simulink model "ANN_Simulation"  (R2024a)
settings: Solver=VariableStepAuto  StartTime=0.0  StopTime=5  RelTol=1e-3
undefined symbols (not defined in the file or in its folder): B, J, Ls, p, Rs, samplingTime, Sm
libraries: slpidlib x1
settings Model: Creator=anugr  LastModifiedBy=anugr
settings DataIOCC: ReturnWorkspaceOutputs=off

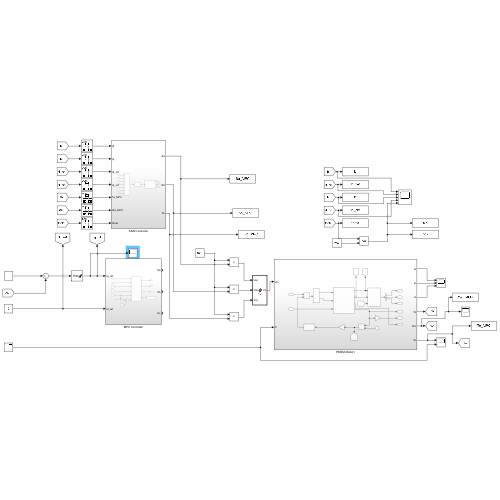
[thumbnail: Simulink's stored preview of the top-level diagram]
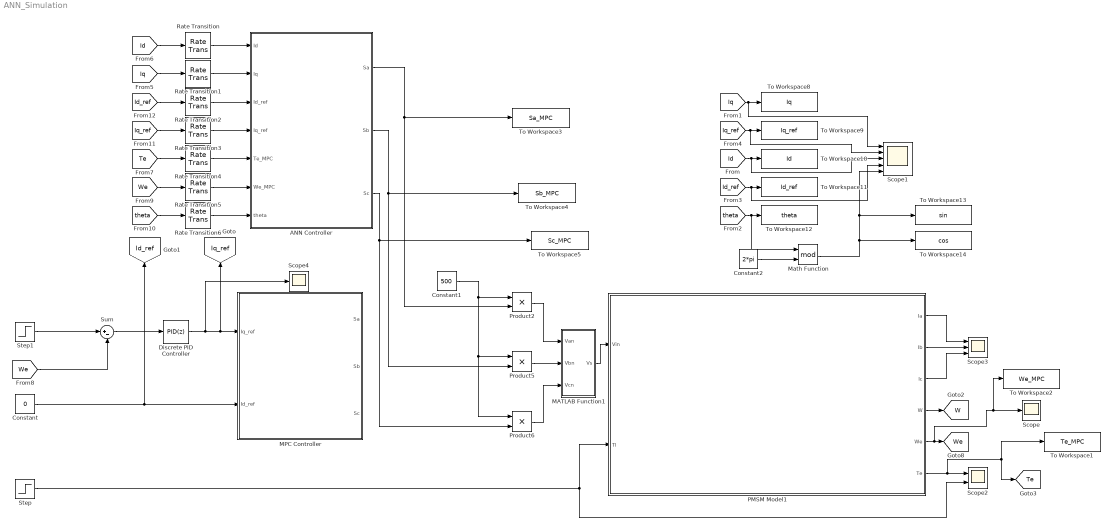
== system ANN_Simulation ==
  ANN Controller : Subsystem
  Constant : Constant  Value=0
  Constant1 : Constant  Value=500
  Constant2 : Constant  Value=2*pi
  Discrete PID Controller : slpidlib/PID Controller  Controller=PID  Form=Parallel  TimeDomain=Discrete-time  UseExternalTs=off  SampleTime=-1  IntegratorMethod=Forward Euler  FilterMethod=Forward Euler  ControllerParametersSource=internal  P=10  I=1  UseKiTs=off  D=1  UseExternalDerivativeSource=off  N=100  UseFilter=on  TunerSelectOption=Transfer Function Based (PID Tuner App)  InitialConditionSource=internal  InitialConditionForIntegrator=0  InitialConditionForFilter=0  DifferentiatorICPrevScaledInput=0  ExternalReset=none  TrackingMode=off  Kt=1  LimitOutput=on  SatLimitsSource=internal  UpperSaturationLimit=20  LowerSaturationLimit=-20  LinearizeAsGain=on  AntiWindupMode=clamping  Kb=1  LimitIntegrator=off  UpperIntegratorSaturationLimit=inf  LowerIntegratorSaturationLimit=-inf  POutMin=[]  POutMax=[]  IOutMin=[]  IOutMax=[]  DOutMin=[]  DOutMax=[]  NOutMin=[]  NOutMax=[]  SumOutMin=[]  SumOutMax=[]  SaturationOutMin=[]  SaturationOutMax=[]  PParamMin=[]  PParamMax=[]  IParamMin=[]  IParamMax=[]  DParamMin=[]  DParamMax=[]  NParamMin=[]  NParamMax=[]  KbParamMin=[]  KbParamMax=[]  KtParamMin=[]  KtParamMax=[]  KbOutMin=[]  KbOutMax=[]  KtOutMin=[]  KtOutMax=[]  IntegratorOutMin=[]  IntegratorOutMax=[]  FilterOutMin=[]  FilterOutMax=[]  SumI1OutMin=[]  SumI1OutMax=[]  SumI2OutMin=[]  SumI2OutMax=[]  SumI3OutMin=[]  SumI3OutMax=[]  SumI4OutMin=[]  SumI4OutMax=[]  SumDOutMin=[]  SumDOutMax=[]  DifferentiatorOutMin=[]  DifferentiatorOutMax=[]  FilterDiffOutCoefMin=[]  FilterDiffOutCoefMax=[]  ReciprocalOutMin=[]  ReciprocalOutMax=[]  SumDenOutMin=[]  SumDenOutMax=[]  SumNumOutMin=[]  SumNumOutMax=[]  DivideOutMin=[]  DivideOutMax=[]  UdiffTsProdOutMin=[]  UdiffTsProdOutMax=[]  NTsProdOutMin=[]  NTsProdOutMax=[]  UintegralTsProdOutMin=[]  UintegralTsProdOutMax=[]  UngainTsProdOutMin=[]  UngainTsProdOutMax=[]  ClampingZeroOutDataTypeStr=Inherit: Inherit via back propagation  ClampingZeroOutMin=[]  ClampingZeroOutMax=[]  FilterDenConstantOutDataTypeStr=Inherit: Inherit via back propagation  FilterDenConstantOutMin=[]  FilterDenConstantOutMax=[]  PCopyOutDataTypeStr=Inherit: Inherit via back propagation  PCopyOutMin=[]  PCopyOutMax=[]  NCopyOutDataTypeStr=Inherit: Inherit via back propagation  NCopyOutMin=[]  NCopyOutMax=[]  IntegratorContinuousStateAttributes=''  IntegratorStateMustResolveToSignalObject=off  IntegratorRTWStateStorageClass=Auto  FilterContinuousStateAttributes=''  FilterStateMustResolveToSignalObject=off  FilterRTWStateStorageClass=Auto  ParallelPVariant=InternalParameters  IdealPVariant=Disabled  IVariant=InternalParameters  DVariant=InternalParameters  IntegratorVariant=Discrete  SatVariant=Enabled  AWVariant=DiscClampingParallel  PCopyVariant=Disabled  TRVariant=Disabled  FdbkBlocksVariant=Forward  IdealPFdbkVariant=Disabled  SatFdbkVariant=Disabled  DerivativeFilterVariant=ForwardEulerFilter  NVariant=InternalParameters  NCopyVariant=Disabled  FilterICVariant=InternalICsFilter  IntegratorICVariant=InternalICs  ExternalResetVariant=Disabled  TRSumVariant=Passthrough  SumFdbkVariant=Disabled  SumVariant=Sum_PID  TsampFilterVariant=InternalTs  TsampNgainVariant=Passthrough  TsampIntegralVariant=Disabled_SignalSpec  ExternalSaturationOutDataTypeStr=Inherit: Same as second input  DerivativeSourceVariant=ErrorSignal
  MATLAB Function1 : MATLAB Function  TreatAsAtomicUnit=on
  MPC Controller : Subsystem
  Math Function : Math  Operator=mod
  PMSM Model1 : Subsystem
  Product2 : Product
  Product5 : Product
  Product6 : Product
  Rate Transition{,1..6} (7 alike) : RateTransition  OutPortSampleTime=5e-5
  Scope : Scope
  Scope1 : Scope  NumInputPorts=5
  Scope2 : Scope  NumInputPorts=2
  Scope3 : Scope  NumInputPorts=3
  Scope4 : Scope
  Step : Step  Time=2.5  After=5  SampleTime=0
  Step1 : Step  Time=0  After=200  SampleTime=0
  Sum : Sum  Inputs=|+-
  To Workspace1 : ToWorkspace  VariableName=Te_MPC  SampleTime=samplingTime*1e-6
      settings: Save2DSignal=2-D array (concatenate along first dimension)
  To Workspace10 : ToWorkspace  VariableName=Id  SampleTime=samplingTime*1e-6
      settings: Save2DSignal=2-D array (concatenate along first dimension)
  To Workspace11 : ToWorkspace  VariableName=Id_ref  SampleTime=samplingTime*1e-6
      settings: Save2DSignal=2-D array (concatenate along first dimension)
  To Workspace12 : ToWorkspace  VariableName=theta  SampleTime=samplingTime*1e-6
      settings: Save2DSignal=2-D array (concatenate along first dimension)
  To Workspace13 : ToWorkspace  VariableName=sin  SampleTime=samplingTime*1e-6
      settings: Save2DSignal=2-D array (concatenate along first dimension)
  To Workspace14 : ToWorkspace  VariableName=cos  SampleTime=samplingTime*1e-6
      settings: Save2DSignal=2-D array (concatenate along first dimension)
  To Workspace2 : ToWorkspace  VariableName=We_MPC  SampleTime=samplingTime*1e-6
      settings: Save2DSignal=2-D array (concatenate along first dimension)
  To Workspace3 : ToWorkspace  VariableName=Sa_MPC  SampleTime=samplingTime*1e-6
      settings: Save2DSignal=2-D array (concatenate along first dimension)
  To Workspace4 : ToWorkspace  VariableName=Sb_MPC  SampleTime=samplingTime*1e-6
      settings: Save2DSignal=2-D array (concatenate along first dimension)
  To Workspace5 : ToWorkspace  VariableName=Sc_MPC  SampleTime=samplingTime*1e-6
      settings: Save2DSignal=2-D array (concatenate along first dimension)
  To Workspace8 : ToWorkspace  VariableName=Iq  SampleTime=samplingTime*1e-6
      settings: Save2DSignal=2-D array (concatenate along first dimension)
  To Workspace9 : ToWorkspace  VariableName=Iq_ref  SampleTime=samplingTime*1e-6
      settings: Save2DSignal=2-D array (concatenate along first dimension)
  tag scope: Id_ref=global, Iq_ref=global, Te=global, W=global, We=global
  wires:
  [Iq_ref] -> Scope1/2, To Workspace9/1
  [Id] -> Scope1/3, To Workspace10/1
  Product6/1 -> MATLAB Function1/3(Vcn)
  Product5/1 -> MATLAB Function1/2(Vbn)
  Math Function/1 -> To Workspace14/1, To Workspace13/1, Scope1/5
  Constant2/1 -> Math Function/2
  PMSM Model1/2(Ib) -> Scope3/2
  Product2/1 -> MATLAB Function1/1(Van)
  PMSM Model1/1(Ia) -> Scope3/1
  PMSM Model1/5(We) -> To Workspace2/1, Scope/1, [We]
  [Iq] -> Scope1/1, To Workspace8/1
  [Id_ref] -> Scope1/4, To Workspace11/1
  [theta] -> Math Function/1, To Workspace12/1
  Sum/1 -> Discrete PID Controller/1
  Step1/1 -> Sum/1
  Discrete PID Controller/1 -> Scope4/1, [Iq_ref], MPC Controller/1(Iq_ref)
  Constant1/1 -> Product5/1, Product6/1, Product2/1
  PMSM Model1/4(W) -> [W]
  [We] -> Sum/2
  PMSM Model1/6(Te) -> To Workspace1/1, [Te], Scope2/1
  Constant/1 -> [Id_ref], MPC Controller/2(Id_ref)
  MATLAB Function1/1(Vs) -> PMSM Model1/1(Vin)
  Step/1 -> Scope2/2, PMSM Model1/2(Tl)
  PMSM Model1/3(Ic) -> Scope3/3
  [Iq] -> Rate Transition1/1
  [Id] -> Rate Transition/1
  [Te] -> Rate Transition4/1
  [We] -> Rate Transition5/1
  [theta] -> Rate Transition6/1
  [Iq_ref] -> Rate Transition3/1
  [Id_ref] -> Rate Transition2/1
  ANN Controller/1(Sa) -> Product2/2, To Workspace3/1
  ANN Controller/2(Sb) -> To Workspace4/1, Product5/2
  ANN Controller/3(Sc) -> Product6/2, To Workspace5/1
  Rate Transition/1 -> ANN Controller/1(Id)
  Rate Transition1/1 -> ANN Controller/2(Iq)
  Rate Transition2/1 -> ANN Controller/3(Id_ref)
  Rate Transition3/1 -> ANN Controller/4(Iq_ref)
  Rate Transition4/1 -> ANN Controller/5(Te_MPC)
  Rate Transition5/1 -> ANN Controller/6(We_MPC)
  Rate Transition6/1 -> ANN Controller/7(theta)

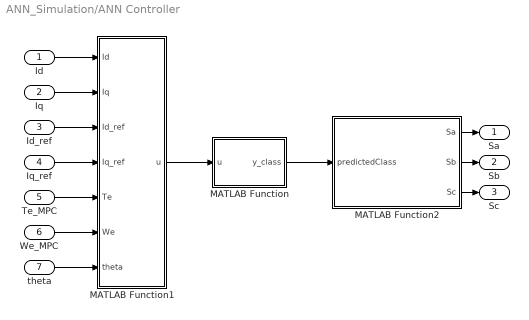
== system ANN_Simulation/ANN Controller ==
  Id : Inport
  Iq : Inport  Port=2
  Id_ref : Inport  Port=3
  Iq_ref : Inport  Port=4
  Te_MPC : Inport  Port=5
  We_MPC : Inport  Port=6
  theta : Inport  Port=7
  MATLAB Function : MATLAB Function  TreatAsAtomicUnit=on
  MATLAB Function1 : MATLAB Function  TreatAsAtomicUnit=on
  MATLAB Function2 : MATLAB Function  TreatAsAtomicUnit=on
  Sa : Outport
  Sb : Outport  Port=2
  Sc : Outport  Port=3
  wires:
  MATLAB Function2/3(Sc) -> Sc/1
  We_MPC/1 -> MATLAB Function1/6(We)
  Iq/1 -> MATLAB Function1/2(Iq)
  MATLAB Function2/1(Sa) -> Sa/1
  MATLAB Function/1(y_class) -> MATLAB Function2/1(predictedClass)
  theta/1 -> MATLAB Function1/7(theta)
  MATLAB Function1/1(u) -> MATLAB Function/1(u)
  Id/1 -> MATLAB Function1/1(Id)
  Te_MPC/1 -> MATLAB Function1/5(Te)
  MATLAB Function2/2(Sb) -> Sb/1
  Id_ref/1 -> MATLAB Function1/3(Id_ref)
  Iq_ref/1 -> MATLAB Function1/4(Iq_ref)

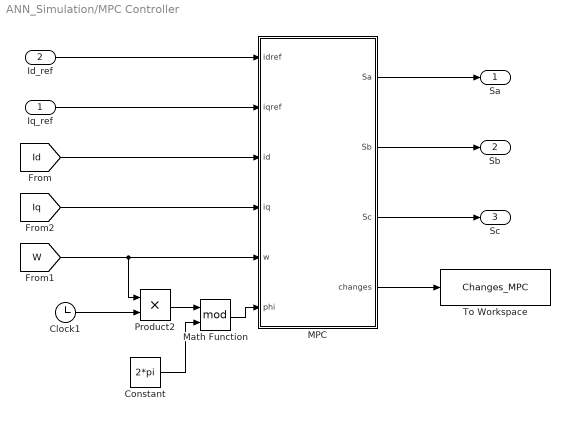
== system ANN_Simulation/MPC Controller ==
  Iq_ref : Inport
  Id_ref : Inport  Port=2
  Clock1 : Clock
  Constant : Constant  Value=2*pi
  MPC : MATLAB Function  TreatAsAtomicUnit=on
  Math Function : Math  Operator=mod
  Product2 : Product
  To Workspace : ToWorkspace  VariableName=Changes_MPC  SaveFormat=Timeseries  SampleTime=-1
  Sa : Outport
  Sb : Outport  Port=2
  Sc : Outport  Port=3
  wires:
  [Iq] -> MPC/4(iq)
  [W] -> MPC/5(w), Product2/1
  MPC/3(Sc) -> Sc/1
  [Id] -> MPC/3(id)
  Id_ref/1 -> MPC/1(idref)
  Iq_ref/1 -> MPC/2(iqref)
  Clock1/1 -> Product2/2
  MPC/2(Sb) -> Sb/1
  MPC/1(Sa) -> Sa/1
  MPC/4(changes) -> To Workspace/1
  Product2/1 -> Math Function/1
  Math Function/1 -> MPC/6(phi)
  Constant/1 -> Math Function/2

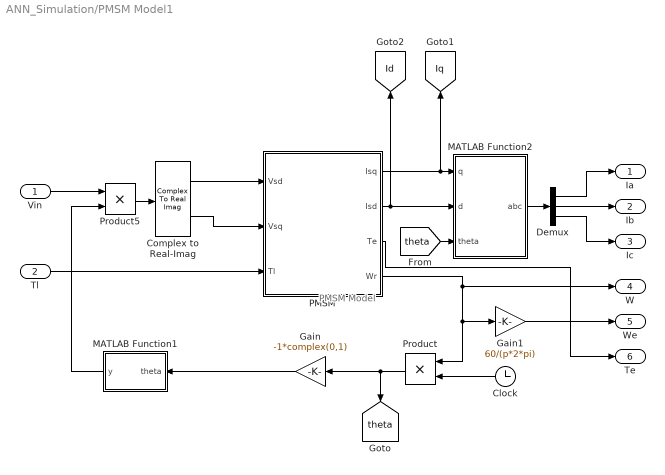
== system ANN_Simulation/PMSM Model1 ==
  note: PMSM Model
  Vin : Inport
  Tl : Inport  Port=2
  Clock : Clock
  Complex to Real-Imag : ComplexToRealImag
  Demux : Demux  Outputs=3
  Gain : Gain  Gain=-1*complex(0,1)
  Gain1 : Gain  Gain=60/(p*2*pi)
  MATLAB Function1 : MATLAB Function  TreatAsAtomicUnit=on
  MATLAB Function2 : MATLAB Function  TreatAsAtomicUnit=on
  PMSM : Subsystem
  Product : Product
  Product5 : Product
  Ia : Outport
  Ib : Outport  Port=2
  Ic : Outport  Port=3
  W : Outport  Port=4
  We : Outport  Port=5
  Te : Outport  Port=6
  tag scope: Id=global, Iq=global, theta=global
  wires:
  Tl/1 -> PMSM/3(Tl)
  PMSM/4(Wr) -> W/1, Gain1/1, Product/1
  Product/1 -> Gain/1, [theta]
  Demux/3 -> Ic/1
  Clock/1 -> Product/2
  PMSM/1(Isq) -> [Iq], MATLAB Function2/1(q)
  MATLAB Function1/1(y) -> Product5/2
  Complex to Real-Imag/1 -> PMSM/1(Vsd)
  PMSM/3(Te) -> Te/1
  PMSM/2(Isd) -> MATLAB Function2/2(d), [Id]
  Complex to Real-Imag/2 -> PMSM/2(Vsq)
  Product5/1 -> Complex to Real-Imag/1
  Gain/1 -> MATLAB Function1/1(theta)
  Demux/1 -> Ia/1
  MATLAB Function2/1(abc) -> Demux/1
  Vin/1 -> Product5/1
  Gain1/1 -> We/1
  Demux/2 -> Ib/1
  [theta] -> MATLAB Function2/3(theta)

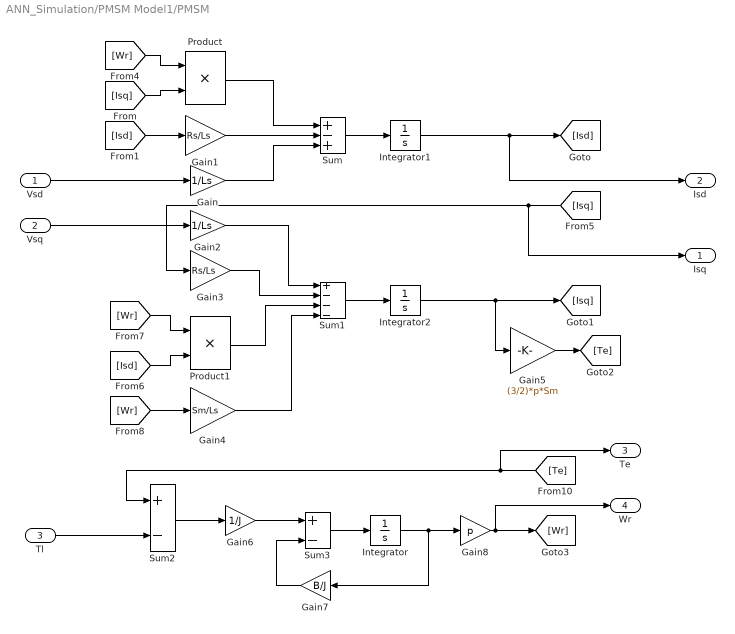
== system ANN_Simulation/PMSM Model1/PMSM ==
  Vsd : Inport
  Vsq : Inport  Port=2
  Tl : Inport  Port=3
  Gain : Gain  Gain=1/Ls
  Gain1 : Gain  Gain=Rs/Ls
  Gain2 : Gain  Gain=1/Ls
  Gain3 : Gain  Gain=Rs/Ls
  Gain4 : Gain  Gain=Sm/Ls
  Gain5 : Gain  Gain=(3/2)*p*Sm
  Gain6 : Gain  Gain=1/J
  Gain7 : Gain  Gain=B/J
  Gain8 : Gain  Gain=p
  Integrator : Integrator
  Integrator1 : Integrator
  Integrator2 : Integrator
  Product : Product
  Product1 : Product
  Sum : Sum  Inputs=+-+
  Sum1 : Sum  Inputs=+---
  Sum2 : Sum  Inputs=+-
  Sum3 : Sum  Inputs=+-
  Isq : Outport
  Isd : Outport  Port=2
  Te : Outport  Port=3
  Wr : Outport  Port=4
  wires:
  Gain5/1 -> [Te]
  [Wr] -> Gain4/1
  [Isq] -> Isq/1, Gain3/1
  [Te] -> Te/1, Sum2/1
  Integrator2/1 -> Gain5/1, [Isq]
  Gain6/1 -> Sum3/1
  Sum1/1 -> Integrator2/1
  Gain/1 -> Sum/3
  Integrator/1 -> Gain8/1, Gain7/1
  Tl/1 -> Sum2/2
  Gain8/1 -> Wr/1, [Wr]
  Gain2/1 -> Sum1/1
  Sum3/1 -> Integrator/1
  Vsd/1 -> Gain/1
  Sum2/1 -> Gain6/1
  [Isd] -> Product1/2
  Gain7/1 -> Sum3/2
  Gain3/1 -> Sum1/2
  Gain4/1 -> Sum1/4
  [Wr] -> Product/1
  [Isq] -> Product/2
  Product1/1 -> Sum1/3
  [Wr] -> Product1/1
  Product/1 -> Sum/1
  Gain1/1 -> Sum/2
  [Isd] -> Gain1/1
  Sum/1 -> Integrator1/1
  Vsq/1 -> Gain2/1
  Integrator1/1 -> Isd/1, [Isd]

== matlab function ANN_Simulation/ANN Controller/MATLAB Function1 ==
  data: Id input; u output; Iq input; Id_ref input; Iq_ref input; Te input; We input; theta input
function u = createANNInputs(Id, Iq, Id_ref, Iq_ref, Te, We, theta)
%#codegen
sinTheta = sin(theta);
cosTheta = cos(theta);
u = [Id; Iq; Id_ref; Iq_ref; Te; We; theta; sinTheta; cosTheta];
end

== matlab function ANN_Simulation/ANN Controller/MATLAB Function ==
  data: u input; y_class output
function y_class = runANN(u)
%#codegen
y = myANNFcn(u);         % ANN raw output (numClasses × 1)
[~, idx] = max(y);       % pick highest activation
y_class = idx - 1;       % convert to class label (0–7)
end

== matlab function ANN_Simulation/ANN Controller/MATLAB Function2 ==
  data: predictedClass input; Sa output; Sb output; Sc output
function [Sa, Sb, Sc] = classToSwitching(predictedClass)
%CLASSTOSWITCHING Converts ANN class output to 3-phase switching signals
%   Input:
%       predictedClass - scalar, integer class (0 to 7)
%   Outputs:
%       Sa, Sb, Sc    - switching signals (0 or 1)

    switch predictedClass
        case 0
            Sa = 0; Sb = 0; Sc = 0;
        case 1
            Sa = 1; Sb = 0; Sc = 0;
        case 2
            Sa = 1; Sb = 1; Sc = 0;
        case 3
            Sa = 0; Sb = 1; Sc = 0;
        case 4
            Sa = 0; Sb = 1; Sc = 1;
        case 5
            Sa = 0; Sb = 0; Sc = 1;
        case 6
            Sa = 1; Sb = 0; Sc = 1;
        case 7
            Sa = 1; Sb = 1; Sc = 1;
        otherwise
            error('Invalid class. Must be an integer from 0 to 7.');
    end
end

== matlab function ANN_Simulation/MPC Controller/MPC ==
  settings: updateMethod=DISCRETE
  data: idref input; Sa output; iqref input; id input; iq input; w input; Sb output; Sc output; phi input; changes output
function [Sa, Sb, Sc, changes] = mpc(idref, iqref, id, iq, w,phi) 
    %% Initialisation 
    R = 0.02;
    Ls = 0.4;
    Vdc = 400;
    Lambda_f = 0.2205;
    Ts = 1e-6;
    imax=80;
    p=4;
    cost=1e14; 
    persistent state; 
    if isempty(state) 
        state = 1; 
    end
    S = [0 0 0; 1 0 0; 1 1 0; 0 1 0; 0 1 1; 0 0 1; 1 0 1; 1 1 1]; 
    prev_state = state;
    for i=1:8
    ud = Vdc*(2/3)*(S(i,1)*cos(phi) + S(i,2)*cos(phi-2*pi/3) + S(i,3)*cos(phi + 2*pi/3)); 
    uq = Vdc*(2/3)* (-S(i,1) *sin(phi) - S(i,2)*sin(phi- 2*pi/3) - S(i,3)*sin(phi + 2*pi/3));
    id1 = ((1 -(R*Ts)/Ls)*id) + ((Ts*ud)/Ls) + (w*Ts*iq) ; 
    iq1 = ((1 - (R*Ts)/Ls)*iq) + ((Ts*uq)/Ls) - ((w*Ts*id)) - (((w*Ts*Lambda_f)/Ls)); 
    f = 0; 
    if abs(id1) > imax || abs(iq1) > imax 
        f = 1e14; 
    end
    current_cost=(idref-id1)^2 + (iqref-iq1)^2 +f; 
    if(current_cost<cost) 
        state=i;
        cost=current_cost;
    end
          
    end
    changes = sum(S(state,:) ~= S(prev_state,:));
    Sa = S(state,1);
    Sb = S(state,2); 
    Sc = S(state,3);
end

== matlab function ANN_Simulation/MATLAB Function1 ==
  data: Van input; Vs output; Vbn input; Vcn input
function Vs = fcn(Van,Vbn,Vcn)

a=complex(cos(2*pi/3),sin(2*pi/3)); 
Vs =(2/3)*(Van+(a*Vbn)+((a^2)*Vcn)) ;

== matlab function ANN_Simulation/PMSM Model1/MATLAB Function1 ==
  data: theta input; y output
function y = fcn(theta)

y = exp((theta));

== matlab function ANN_Simulation/PMSM Model1/MATLAB Function2 ==
  data: q input; d input; abc output; theta input
function abc = dq_to_abc(q, d, theta)
    % Inputs:
    % d, q   : DQ components
    % theta  : Electrical angle in radians

    % Transformation matrix
    T = [cos(theta), -sin(theta), 1; 
         cos(theta - 2*pi/3), -sin(theta - 2*pi/3), 1; 
         cos(theta + 2*pi/3), -sin(theta + 2*pi/3), 1];

    % Calculate abc components
    abc = (2/3) * T * [d; q; 0];
end
